simulink model "stp2_2"  (R2016b)
settings: Solver=VariableStepAuto  StartTime=0.0  StopTime=10.0  RelTol=1e-3
undefined symbols (not defined in the file): Ad2, Bd2
settings Model: Creator=arq  LastModifiedBy=arq

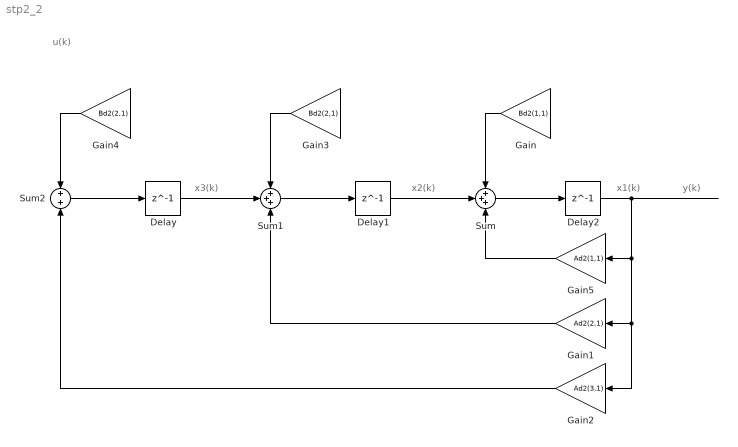
== system stp2_2 ==
  note: u(k)
  note: x3(k)
  note: x2(k)
  note: x1(k)
  note: y(k)
  Delay : Delay  DelayLength=1  InitialCondition=0
  Delay1 : Delay  DelayLength=1  InitialCondition=0
  Delay2 : Delay  DelayLength=1  InitialCondition=0
  Gain : Gain  Gain=Bd2(1,1)
  Gain1 : Gain  Gain=Ad2(2,1)
  Gain2 : Gain  Gain=Ad2(3,1)
  Gain3 : Gain  Gain=Bd2(2,1)
  Gain4 : Gain  Gain=Bd2(2,1)
  Gain5 : Gain  Gain=Ad2(1,1)
  Sum : Sum  Inputs=3
  Sum1 : Sum  Inputs=3
  Sum2 : Sum  Inputs=2
  wires:
  Delay2/1 -> Gain2/1, Gain1/1, Gain5/1
  ? -> Gain/1, Gain3/1, Gain4/1
  Delay1/1 -> Sum/2
  Sum/1 -> Delay2/1
  Sum1/1 -> Delay1/1
  Delay/1 -> Sum1/2
  Gain5/1 -> Sum/3
  Gain1/1 -> Sum1/3
  Gain2/1 -> Sum2/2
  Sum2/1 -> Delay/1
  Gain/1 -> Sum/1
  Gain3/1 -> Sum1/1
  Gain4/1 -> Sum2/1
